simulink model "lab_three_task_two"  (R2018b)
settings: Solver=VariableStepAuto  StartTime=0.0  StopTime=10.0  RelTol=1e-3
settings Model: Creator=Romario  LastModifiedBy=Romario

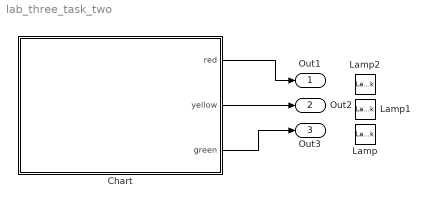
== system lab_three_task_two ==
  Chart : Stateflow chart  TreatAsAtomicUnit=on
  Lamp : LampBlock  WebBlockId=2  LabelPosition=Hide
  Lamp1 : LampBlock  WebBlockId=3  LabelPosition=Hide
  Lamp2 : LampBlock  WebBlockId=4  LabelPosition=Hide
  Out1 : Outport
  Out2 : Outport  Port=2
  Out3 : Outport  Port=3
  wires:
  Chart/1(red) -> Out1/1
  Chart/2(yellow) -> Out2/1
  Chart/3(green) -> Out3/1

== stateflow chart lab_three_task_two/Chart ==
  state YellowLed
    en:
    red=0;
    green=0;
    yellow=1;
    du:
    ex:
  state RedLed
    en:
    red=1;
    green=0;
    yellow=0;
    du:
    ex:
  state GreenLed
    en:
    red=0;
    green=1;
    yellow=0;
    du:
    ex:
  (default) -> RedLed
  RedLed -> YellowLed : [after(3,sec)]
  GreenLed -> RedLed : [after(3,sec)]
  YellowLed -> GreenLed : [after(3,sec)]
  data: red output uint8; yellow output uint8; green output uint8
